simulink model "relay_trial"  (R2017a)
settings: Solver=ode45  StartTime=0.0  StopTime=50  MaxStep=1e-3  RelTol=1e-3  EnableMultiTasking=on
libraries: simulink x31, powerlib_extras x1, cstblocks x1
settings Model: Creator=jmgomes  LastModifiedBy=guir
settings DataIOCC: SaveFormat=Array  SignalLoggingSaveFormat=ModelDataLogs
settings OptimizationCC: ExpressionDepthLimit=2147483647  InitFltsAndDblsToZero=on  LifeSpan=inf
settings DebuggingCC: SaveWithParameterizedLinksMsg=none  UnderspecifiedInitializationDetection=Classic  MergeDetectMultiDrivingBlocksExec=none  SignalResolutionControl=TryResolveAllWithWarning  SolverPrmCheckMsg=warning  MultiTaskDSMMsg=warning  MultiTaskCondExecSysMsg=none  FcnCallInpInsideContextMsg=warning  StateNameClashWarn=warning  SFUnexpectedBacktrackingDiag=warning  SFNoUnconditionalDefaultTransitionDiag=warning  SFExecutionAtInitializationDiag=none
settings HardwareCC: ProdBitPerPointer=32  ProdBitPerSizeT=32  ProdBitPerPtrDiffT=32  ProdLargestAtomicFloat=None  ProdIntDivRoundTo=Undefined  ProdEndianess=Unspecified  ProdWordSize=32  ProdHWDeviceType=32-bit Generic
settings ModelReferenceCC: PropagateSignalLabelsOutOfModel=off
settings GRTTargetCC: TargetFcnLib=ansi_tfl_tmw.mat  TargetLangStandard=C89/C90 (ANSI)  GeneratePreprocessorConditionals=Disable all  CombineOutputUpdateFcns=off  GRTInterface=on
settings ConfigComp: CovMetricSettings=dw  CovHtmlReporting=on  CovSaveCumulativeToWorkspaceVar=on  CovSaveSingleToWorkspaceVar=on  CovExternalEMLEnable=off

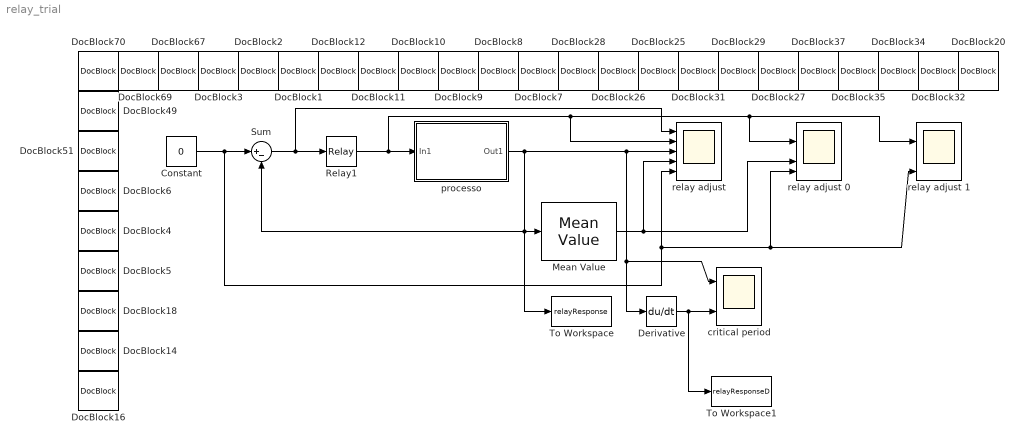
== system relay_trial ==
  Constant : Constant  Value=0
  Derivative : Derivative
  DocBlock{1..12,14,16,18,20,25..29,31..32,34..35,37,49,51,67,69..70} (31 alike) : simulink/Model-Wide Utilities/DocBlock  DocumentType=Text
      content=|
      | Type your documentation here
  Mean Value : powerlib_extras/Measurements/Mean Value  Period=pi
  Relay1 : Relay  OnSwitchValue=1  OffSwitchValue=-1  OnOutputValue=0.02  OffOutputValue=-0.02
  Sum : Sum  Inputs=|+-
  To Workspace : ToWorkspace  VariableName=relayResponse  SampleTime=-1
  To Workspace1 : ToWorkspace  VariableName=relayResponseD  SampleTime=-1
  critical period : Scope  NumInputPorts=2
  processo : Subsystem
  relay adjust : Scope  NumInputPorts=5
  relay adjust 0 : Scope  NumInputPorts=5
  relay adjust 1 : Scope  NumInputPorts=5
  wires:
  Relay1/1 -> processo/1(In1), relay adjust 1/2, relay adjust 0/2, relay adjust/2
  Sum/1 -> Relay1/1, relay adjust/1
  Constant/1 -> relay adjust 1/5, relay adjust 0/5, relay adjust/5, Sum/1
  processo/1(Out1) -> To Workspace/1, Sum/2, Mean Value/1, relay adjust/3, Derivative/1, critical period/1
  Mean Value/1 -> relay adjust 0/4, relay adjust/4
  Derivative/1 -> critical period/2, To Workspace1/1

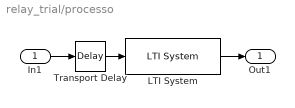
== system relay_trial/processo ==
  In1 : Inport
  LTI System : cstblocks/LTI System  sys=tfr  IC=[]
  Transport Delay : TransportDelay  DelayTime=0.34
  Out1 : Outport
  wires:
  In1/1 -> Transport Delay/1
  Transport Delay/1 -> LTI System/1
  LTI System/1 -> Out1/1
